simulink model "MultiInverter_StrongGridInstability_Simulation"  (R2020b)
settings: Solver=FixedStepAuto  StartTime=0  StopTime=2  FixedStep=Ts  RelTol=1e-3
undefined symbols (not defined in the file): DeviceDiscreDamping, DevicePara, DeviceType, Fbase, OtherInputs, PowerFlow, Sbase, Ts, Vbase, Wbase, x_e, Ybase, Zbase
libraries: powerlib x61, SimplexPS x21
settings Model: Creator=admin_user  LastModifiedBy=admin_user
settings DataIOCC: ReturnWorkspaceOutputs=off

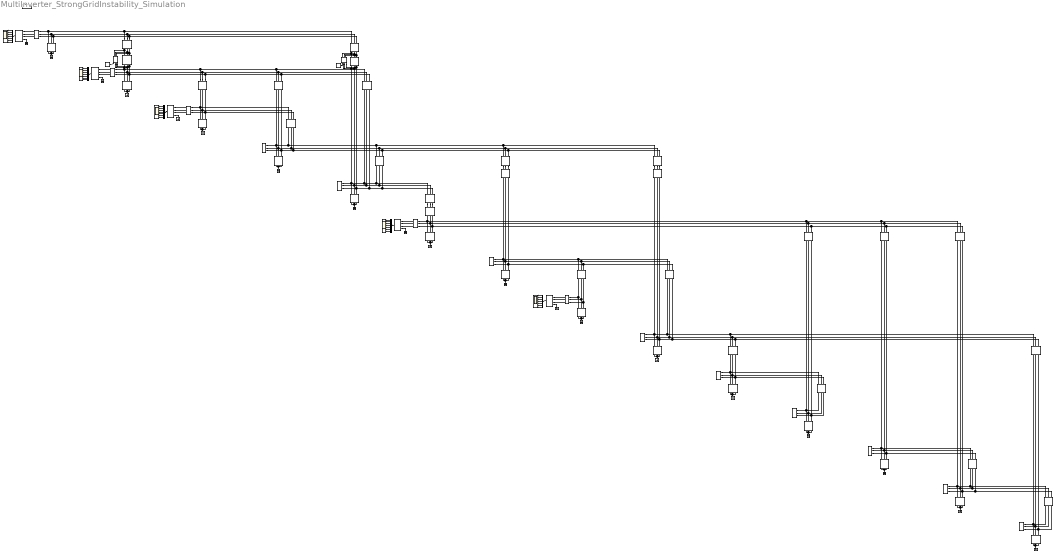
== system MultiInverter_StrongGridInstability_Simulation ==
  B-GND{1,4,8,10,14,16,20,23..24,27,29..30,32,34} (14 alike) : powerlib/Elements/Ground  LConnTagsString=a
  Branch1010 : powerlib/Elements/Three-Phase Parallel RLC Branch  LConnTagsString=A|B|C  RConnTagsString=A|B|C  BranchType=RLC  Resistance=(11.8667)*Zbase  Inductance=(18.4139)*Zbase/Wbase  Capacitance=(1e-05)*Ybase/Wbase  Measurements=None
      settings: SourceProductBaseCode=PS
  Branch1011 : powerlib/Elements/Three-Phase Series RLC Branch  LConnTagsString=A|B|C  RConnTagsString=A|B|C  BranchType=RL  Resistance=(0.08205)*Zbase  Inductance=(0.19207)*Zbase/Wbase  Capacitance=1e-6  Measurements=None
  Branch11 : powerlib/Elements/Three-Phase Parallel RLC Branch  LConnTagsString=A|B|C  RConnTagsString=A|B|C  BranchType=C  Resistance=(Inf)*Zbase  Inductance=1e-3  Capacitance=(0.102)*Ybase/Wbase  Measurements=None
      settings: SourceProductBaseCode=PS
  Branch1111 : powerlib/Elements/Three-Phase Parallel RLC Branch  LConnTagsString=A|B|C  RConnTagsString=A|B|C  BranchType=RLC  Resistance=(31.8511)*Zbase  Inductance=(61.9328)*Zbase/Wbase  Capacitance=(1e-05)*Ybase/Wbase  Measurements=None
      settings: SourceProductBaseCode=PS
  Branch12 : powerlib/Elements/Three-Phase Series RLC Branch  LConnTagsString=A|B|C  RConnTagsString=A|B|C  BranchType=RL  Resistance=(0.01938)*Zbase/5  Inductance=(0.05917)*Zbase/Wbase/5  Capacitance=1e-6  Measurements=None
  Branch1212 : powerlib/Elements/Three-Phase Parallel RLC Branch  LConnTagsString=A|B|C  RConnTagsString=A|B|C  BranchType=RLC  Resistance=(18.8878)*Zbase  Inductance=(72.0098)*Zbase/Wbase  Capacitance=(1e-05)*Ybase/Wbase  Measurements=None
      settings: SourceProductBaseCode=PS
  Branch1213 : powerlib/Elements/Three-Phase Series RLC Branch  LConnTagsString=A|B|C  RConnTagsString=A|B|C  BranchType=RL  Resistance=(0.22092)*Zbase  Inductance=(0.19988)*Zbase/Wbase  Capacitance=1e-6  Measurements=None
  Branch12_v1 : powerlib/Elements/Three-Phase Series RLC Branch  LConnTagsString=A|B|C  RConnTagsString=A|B|C  BranchType=RL  Resistance=(0.01938)*Zbase/5*4  Inductance=(0.05917)*Zbase/Wbase/5*4  Capacitance=1e-6  Measurements=None
  Branch1313 : powerlib/Elements/Three-Phase Parallel RLC Branch  LConnTagsString=A|B|C  RConnTagsString=A|B|C  BranchType=RLC  Resistance=(8.2956)*Zbase  Inductance=(19.3087)*Zbase/Wbase  Capacitance=(1e-05)*Ybase/Wbase  Measurements=None
      settings: SourceProductBaseCode=PS
  Branch1314 : powerlib/Elements/Three-Phase Series RLC Branch  LConnTagsString=A|B|C  RConnTagsString=A|B|C  BranchType=RL  Resistance=(0.17093)*Zbase  Inductance=(0.34802)*Zbase/Wbase  Capacitance=1e-6  Measurements=None
  Branch1414 : powerlib/Elements/Three-Phase Parallel RLC Branch  LConnTagsString=A|B|C  RConnTagsString=A|B|C  BranchType=RLC  Resistance=(7.0495)*Zbase  Inductance=(21.0075)*Zbase/Wbase  Capacitance=(1e-05)*Ybase/Wbase  Measurements=None
      settings: SourceProductBaseCode=PS
  Branch15 : powerlib/Elements/Three-Phase Series RLC Branch  LConnTagsString=A|B|C  RConnTagsString=A|B|C  BranchType=RL  Resistance=(0.05403)*Zbase/5  Inductance=(0.22304)*Zbase/Wbase/5  Capacitance=1e-6  Measurements=None
  Branch15_v1 : powerlib/Elements/Three-Phase Series RLC Branch  LConnTagsString=A|B|C  RConnTagsString=A|B|C  BranchType=RL  Resistance=(0.05403)*Zbase/5*4  Inductance=(0.22304)*Zbase/Wbase/5*4  Capacitance=1e-6  Measurements=None
  Branch22 : powerlib/Elements/Three-Phase Parallel RLC Branch  LConnTagsString=A|B|C  RConnTagsString=A|B|C  BranchType=RLC  Resistance=(5.0324)*Zbase  Inductance=(8.5986)*Zbase/Wbase  Capacitance=(0.1652)*Ybase/Wbase  Measurements=None
      settings: SourceProductBaseCode=PS
  Branch23 : powerlib/Elements/Three-Phase Series RLC Branch  LConnTagsString=A|B|C  RConnTagsString=A|B|C  BranchType=RL  Resistance=(0.04699)*Zbase  Inductance=(0.19797)*Zbase/Wbase  Capacitance=1e-6  Measurements=None
  Branch24 : powerlib/Elements/Three-Phase Series RLC Branch  LConnTagsString=A|B|C  RConnTagsString=A|B|C  BranchType=RL  Resistance=(0.05811)*Zbase  Inductance=(0.17632)*Zbase/Wbase  Capacitance=1e-6  Measurements=None
  Branch25 : powerlib/Elements/Three-Phase Series RLC Branch  LConnTagsString=A|B|C  RConnTagsString=A|B|C  BranchType=RL  Resistance=(0.05695)*Zbase  Inductance=(0.17388)*Zbase/Wbase  Capacitance=1e-6  Measurements=None
  Branch33 : powerlib/Elements/Three-Phase Parallel RLC Branch  LConnTagsString=A|B|C  RConnTagsString=A|B|C  BranchType=RLC  Resistance=(1.0829)*Zbase  Inductance=(5.3689)*Zbase/Wbase  Capacitance=(0.0566)*Ybase/Wbase  Measurements=None
      settings: SourceProductBaseCode=PS
  Branch34 : powerlib/Elements/Three-Phase Series RLC Branch  LConnTagsString=A|B|C  RConnTagsString=A|B|C  BranchType=RL  Resistance=(0.06701)*Zbase  Inductance=(0.17103)*Zbase/Wbase  Capacitance=1e-6  Measurements=None
  Branch44 : powerlib/Elements/Three-Phase Parallel RLC Branch  LConnTagsString=A|B|C  RConnTagsString=A|B|C  BranchType=RC  Resistance=(2.196)*Zbase  Inductance=1e-3  Capacitance=(0.083954)*Ybase/Wbase  Measurements=None
      settings: SourceProductBaseCode=PS
  Branch45 : powerlib/Elements/Three-Phase Series RLC Branch  LConnTagsString=A|B|C  RConnTagsString=A|B|C  BranchType=RL  Resistance=(0.01335)*Zbase  Inductance=(0.04211)*Zbase/Wbase  Capacitance=1e-6  Measurements=None
  Branch47 : powerlib/Elements/Three-Phase Series RLC Branch  LConnTagsString=A|B|C  RConnTagsString=A|B|C  BranchType=RL  Resistance=(0.020912)*Zbase  Inductance=(0.20912)*Zbase/Wbase  Capacitance=1e-6  Measurements=None
  Branch49 : powerlib/Elements/Three-Phase Series RLC Branch  LConnTagsString=A|B|C  RConnTagsString=A|B|C  BranchType=RL  Resistance=(0.055618)*Zbase  Inductance=(0.55618)*Zbase/Wbase  Capacitance=1e-6  Measurements=None
  Branch55 : powerlib/Elements/Three-Phase Parallel RLC Branch  LConnTagsString=A|B|C  RConnTagsString=A|B|C  BranchType=RLC  Resistance=(13.9338)*Zbase  Inductance=(66.1856)*Zbase/Wbase  Capacitance=(0.0838)*Ybase/Wbase  Measurements=None
      settings: SourceProductBaseCode=PS
  Branch56 : powerlib/Elements/Three-Phase Series RLC Branch  LConnTagsString=A|B|C  RConnTagsString=A|B|C  BranchType=RL  Resistance=(0.025202)*Zbase  Inductance=(0.25202)*Zbase/Wbase  Capacitance=1e-6  Measurements=None
  Branch611 : powerlib/Elements/Three-Phase Series RLC Branch  LConnTagsString=A|B|C  RConnTagsString=A|B|C  BranchType=RL  Resistance=(0.09498)*Zbase  Inductance=(0.1989)*Zbase/Wbase  Capacitance=1e-6  Measurements=None
  Branch612 : powerlib/Elements/Three-Phase Series RLC Branch  LConnTagsString=A|B|C  RConnTagsString=A|B|C  BranchType=RL  Resistance=(0.12291)*Zbase  Inductance=(0.25581)*Zbase/Wbase  Capacitance=1e-6  Measurements=None
  Branch613 : powerlib/Elements/Three-Phase Series RLC Branch  LConnTagsString=A|B|C  RConnTagsString=A|B|C  BranchType=RL  Resistance=(0.06615)*Zbase  Inductance=(0.13027)*Zbase/Wbase  Capacitance=1e-6  Measurements=None
  Branch66 : powerlib/Elements/Three-Phase Parallel RLC Branch  LConnTagsString=A|B|C  RConnTagsString=A|B|C  BranchType=RLC  Resistance=(10.2223)*Zbase  Inductance=(15.2653)*Zbase/Wbase  Capacitance=(1e-05)*Ybase/Wbase  Measurements=None
      settings: SourceProductBaseCode=PS
  Branch77 : powerlib/Elements/Three-Phase Parallel RLC Branch  LConnTagsString=A|B|C  RConnTagsString=A|B|C  BranchType=C  Resistance=(Inf)*Zbase  Inductance=1e-3  Capacitance=(1e-05)*Ybase/Wbase  Measurements=None
      settings: SourceProductBaseCode=PS
  Branch78 : powerlib/Elements/Three-Phase Series RLC Branch  LConnTagsString=A|B|C  RConnTagsString=A|B|C  BranchType=RL  Resistance=(0.017615)*Zbase  Inductance=(0.17615)*Zbase/Wbase  Capacitance=1e-6  Measurements=None
  Branch79 : powerlib/Elements/Three-Phase Series RLC Branch  LConnTagsString=A|B|C  RConnTagsString=A|B|C  BranchType=RL  Resistance=(0.011001)*Zbase  Inductance=(0.11001)*Zbase/Wbase  Capacitance=1e-6  Measurements=None
  Branch88 : powerlib/Elements/Three-Phase Parallel RLC Branch  LConnTagsString=A|B|C  RConnTagsString=A|B|C  BranchType=C  Resistance=(Inf)*Zbase  Inductance=1e-3  Capacitance=(1e-05)*Ybase/Wbase  Measurements=None
      settings: SourceProductBaseCode=PS
  Branch910 : powerlib/Elements/Three-Phase Series RLC Branch  LConnTagsString=A|B|C  RConnTagsString=A|B|C  BranchType=RL  Resistance=(0.03181)*Zbase  Inductance=(0.0845)*Zbase/Wbase  Capacitance=1e-6  Measurements=None
  Branch914 : powerlib/Elements/Three-Phase Series RLC Branch  LConnTagsString=A|B|C  RConnTagsString=A|B|C  BranchType=RL  Resistance=(0.12711)*Zbase  Inductance=(0.27038)*Zbase/Wbase  Capacitance=1e-6  Measurements=None
  Branch99 : powerlib/Elements/Three-Phase Parallel RLC Branch  LConnTagsString=A|B|C  RConnTagsString=A|B|C  BranchType=RLC  Resistance=(3.6116)*Zbase  Inductance=(6.4182)*Zbase/Wbase  Capacitance=(1e-05)*Ybase/Wbase  Measurements=None
      settings: SourceProductBaseCode=PS
  Bus{1..14} (14 alike) : SimplexPS/Three-Phase Bus  Vbase=1  Sbase=1
      settings: SourceProductName=Simplex Power Systems
  D-GND{1..3,6,8} (5 alike) : powerlib/Elements/Ground  LConnTagsString=a
  D-Scope{1..3,6,8} (5 alike) : Scope  NumInputPorts=7
  DS-Bus{1..3,6,8} (5 alike) : BusSelector  OutputSignals=v_dq,i_dq,v_abc,i_abc,w,theta,pq
  Single Pulse : SimplexPS/Single Pulse  t0=1  dt=0.4  Am=1
      settings: SourceProductName=Simplex Power Systems
  Single Pulse1 : SimplexPS/Single Pulse  t0=1  dt=0.4  Am=1
      settings: SourceProductName=Simplex Power Systems
  Three-Phase Breaker : powerlib/Elements/Three-Phase Breaker  InitialState=open  SwitchA=on  SwitchB=on  SwitchC=on  SwitchTimes="[1/60  5/60]"  External=on  BreakerResistance=0.01  SnubberResistance=1e6  SnubberCapacitance=inf  Measurements=None
  Three-Phase Breaker1 : powerlib/Elements/Three-Phase Breaker  InitialState=open  SwitchA=on  SwitchB=on  SwitchC=on  SwitchTimes="[1/60  5/60]"  External=on  BreakerResistance=0.01  SnubberResistance=1e6  SnubberCapacitance=inf  Measurements=None
  Transformer47 : powerlib/Elements/Three-Phase Transformer (Two Windings)  Winding1Connection=Yg  Winding2Connection=Yg  CoreType=Three single-phase transformers  SetSaturation=off  Hysteresis=off  DataFile='hysteresis'  SetInitialFlux=off  Measurements=None  UNITS=pu  NominalPower=[Sbase, Fbase]  Winding1=[0.978*Vbase, 0, 0]  Winding2=[Vbase, 0, 0]  Rm=1e4  Lm=1e4  L0=0.5  Saturation=[ 0,0 ; 0.0024,1.2 ; 1.0,1.52 ]  InitialFluxes=[ 0.8 , -0.8 , 0.7 ]  BreakLoop=off  DiscreteSolver=Trapezoidal iterative  DataType=off  TransfoNumber=1
  Transformer49 : powerlib/Elements/Three-Phase Transformer (Two Windings)  Winding1Connection=Yg  Winding2Connection=Yg  CoreType=Three single-phase transformers  SetSaturation=off  Hysteresis=off  DataFile='hysteresis'  SetInitialFlux=off  Measurements=None  UNITS=pu  NominalPower=[Sbase, Fbase]  Winding1=[0.969*Vbase, 0, 0]  Winding2=[Vbase, 0, 0]  Rm=1e4  Lm=1e4  L0=0.5  Saturation=[ 0,0 ; 0.0024,1.2 ; 1.0,1.52 ]  InitialFluxes=[ 0.8 , -0.8 , 0.7 ]  BreakLoop=off  DiscreteSolver=Trapezoidal iterative  DataType=off  TransfoNumber=1
  Transformer56 : powerlib/Elements/Three-Phase Transformer (Two Windings)  Winding1Connection=Yg  Winding2Connection=Yg  CoreType=Three single-phase transformers  SetSaturation=off  Hysteresis=off  DataFile='hysteresis'  SetInitialFlux=off  Measurements=None  UNITS=pu  NominalPower=[Sbase, Fbase]  Winding1=[0.932*Vbase, 0, 0]  Winding2=[Vbase, 0, 0]  Rm=1e4  Lm=1e4  L0=0.5  Saturation=[ 0,0 ; 0.0024,1.2 ; 1.0,1.52 ]  InitialFluxes=[ 0.8 , -0.8 , 0.7 ]  BreakLoop=off  DiscreteSolver=Trapezoidal iterative  DataType=off  TransfoNumber=1
  VSI-Droop1 : SimplexPS/Grid-Forming Voltage-Source Inverter (dq-Frame System Object)  Ts=Ts  Sbase=Sbase  Vbase=Vbase  Wbase=Wbase  DeviceType=DeviceType{1}  DevicePara=DevicePara{1}  PowerFlow=PowerFlow{1}  x0=x_e{1}  OtherInputs=OtherInputs{1}  DiscreMethod=Hybrid Trapezoidal  EnableInsideModification=off  DiscreDampingFlag=on  DiscreDampingValue=DeviceDiscreDamping{1}  LinearizationTimes=1  DirectFeedthrough=off
      settings: SourceProductName=Simplex Power Systems
  VSI-Droop3 : SimplexPS/Grid-Forming Voltage-Source Inverter (dq-Frame System Object)  Ts=Ts  Sbase=Sbase  Vbase=Vbase  Wbase=Wbase  DeviceType=DeviceType{3}  DevicePara=DevicePara{3}  PowerFlow=PowerFlow{3}  x0=x_e{3}  OtherInputs=OtherInputs{3}  DiscreMethod=Hybrid Trapezoidal  EnableInsideModification=off  DiscreDampingFlag=on  DiscreDampingValue=DeviceDiscreDamping{3}  LinearizationTimes=1  DirectFeedthrough=off
      settings: SourceProductName=Simplex Power Systems
  VSI-Droop6 : SimplexPS/Grid-Forming Voltage-Source Inverter (dq-Frame System Object)  Ts=Ts  Sbase=Sbase  Vbase=Vbase  Wbase=Wbase  DeviceType=DeviceType{6}  DevicePara=DevicePara{6}  PowerFlow=PowerFlow{6}  x0=x_e{6}  OtherInputs=OtherInputs{6}  DiscreMethod=Hybrid Trapezoidal  EnableInsideModification=off  DiscreDampingFlag=on  DiscreDampingValue=DeviceDiscreDamping{6}  LinearizationTimes=1  DirectFeedthrough=off
      settings: SourceProductName=Simplex Power Systems
  VSI-PLL2 : SimplexPS/Grid-Following Voltage-Source Inverter (dq-Frame System Object)  Ts=Ts  Sbase=Sbase  Vbase=Vbase  Wbase=Wbase  DeviceType=DeviceType{2}  DevicePara=DevicePara{2}  PowerFlow=PowerFlow{2}  x0=x_e{2}  OtherInputs=OtherInputs{2}  DiscreMethod=Hybrid Trapezoidal  EnableInsideModification=off  DiscreDampingFlag=on  DiscreDampingValue=DeviceDiscreDamping{2}  LinearizationTimes=1  DirectFeedthrough=off
      settings: SourceProductName=Simplex Power Systems
  VSI-PLL8 : SimplexPS/Grid-Following Voltage-Source Inverter (dq-Frame System Object)  Ts=Ts  Sbase=Sbase  Vbase=Vbase  Wbase=Wbase  DeviceType=DeviceType{8}  DevicePara=DevicePara{8}  PowerFlow=PowerFlow{8}  x0=x_e{8}  OtherInputs=OtherInputs{8}  DiscreMethod=Hybrid Trapezoidal  EnableInsideModification=off  DiscreDampingFlag=on  DiscreDampingValue=DeviceDiscreDamping{8}  LinearizationTimes=1  DirectFeedthrough=off
      settings: SourceProductName=Simplex Power Systems
  powergui : powerlib/powergui  Priority=1  SimulationMode=Discrete  SampleTime=Ts  frequency=60  Iterations=50  frequencyindice=0  Pbase=100e6  ErrMax=1e-4  UnitsV=kV  UnitsW=MW  buscounter=0  FunctionMessages=off  echomessages=off  EnableUseOfTLC=off  CurrentSourceSwitches=off  DisableSnubberDevices=off  DisableRonSwitches=off  DisableVfSwitches=off  DisplayEquations=off  AutomaticDiscreteSolvers=off  SolverType=Tustin/Backward Euler (TBE)  Interpol=off  ExternalGateDelay=off  methode=off  Ts=100  x0status=blocks  SPID=on  SwTol=0  HookPort=off  NonlinearTolerance=1e-4  nMaxIteration=100  ContinueOnMaxIteration=off  RestoreLinks=warning  ResistiveCurrentMeasurement=off  Frange=[0:2:500]  Ylog=off  Xlog=on  ShowGrid=off  save=off  variable=ZData  structure=0  ZoomFFT=off  StartTime=0.0  cycles=1  DisplayStyle=1  fundamental=60  FreqAxis=off  MaxFrequency=1000  frequencyindicesteady=1  RmsSteady=1  display=off
  wires:
  VSI-Droop1/1 -> DS-Bus1/1
  DS-Bus1/1 -> D-Scope1/1  "<v_dq>"
  DS-Bus1/2 -> D-Scope1/2  "<i_dq>"
  DS-Bus1/3 -> D-Scope1/3  "<v_abc>"
  DS-Bus1/4 -> D-Scope1/4  "<i_abc>"
  DS-Bus1/5 -> D-Scope1/5  "<w>"
  DS-Bus1/6 -> D-Scope1/6  "<theta>"
  DS-Bus1/7 -> D-Scope1/7  "<pq>"
  VSI-PLL2/1 -> DS-Bus2/1
  DS-Bus2/1 -> D-Scope2/1  "<v_dq>"
  DS-Bus2/2 -> D-Scope2/2  "<i_dq>"
  DS-Bus2/3 -> D-Scope2/3  "<v_abc>"
  DS-Bus2/4 -> D-Scope2/4  "<i_abc>"
  DS-Bus2/5 -> D-Scope2/5  "<w>"
  DS-Bus2/6 -> D-Scope2/6  "<theta>"
  DS-Bus2/7 -> D-Scope2/7  "<pq>"
  VSI-Droop3/1 -> DS-Bus3/1
  DS-Bus3/1 -> D-Scope3/1  "<v_dq>"
  DS-Bus3/2 -> D-Scope3/2  "<i_dq>"
  DS-Bus3/3 -> D-Scope3/3  "<v_abc>"
  DS-Bus3/4 -> D-Scope3/4  "<i_abc>"
  DS-Bus3/5 -> D-Scope3/5  "<w>"
  DS-Bus3/6 -> D-Scope3/6  "<theta>"
  DS-Bus3/7 -> D-Scope3/7  "<pq>"
  VSI-Droop6/1 -> DS-Bus6/1
  DS-Bus6/1 -> D-Scope6/1  "<v_dq>"
  DS-Bus6/2 -> D-Scope6/2  "<i_dq>"
  DS-Bus6/3 -> D-Scope6/3  "<v_abc>"
  DS-Bus6/4 -> D-Scope6/4  "<i_abc>"
  DS-Bus6/5 -> D-Scope6/5  "<w>"
  DS-Bus6/6 -> D-Scope6/6  "<theta>"
  DS-Bus6/7 -> D-Scope6/7  "<pq>"
  VSI-PLL8/1 -> DS-Bus8/1
  DS-Bus8/1 -> D-Scope8/1  "<v_dq>"
  DS-Bus8/2 -> D-Scope8/2  "<i_dq>"
  DS-Bus8/3 -> D-Scope8/3  "<v_abc>"
  DS-Bus8/4 -> D-Scope8/4  "<i_abc>"
  DS-Bus8/5 -> D-Scope8/5  "<w>"
  DS-Bus8/6 -> D-Scope8/6  "<theta>"
  DS-Bus8/7 -> D-Scope8/7  "<pq>"
  Single Pulse/1 -> Three-Phase Breaker/1
  Single Pulse1/1 -> Three-Phase Breaker1/1
  connections:
  VSI-Droop1/LConn1 -- Bus1/LConn1
  VSI-Droop1/LConn2 -- Bus1/LConn2
  VSI-Droop1/LConn3 -- Bus1/LConn3
  VSI-PLL2/LConn1 -- Bus2/LConn1
  VSI-PLL2/LConn2 -- Bus2/LConn2
  VSI-PLL2/LConn3 -- Bus2/LConn3
  VSI-Droop3/LConn1 -- Bus3/LConn1
  VSI-Droop3/LConn2 -- Bus3/LConn2
  VSI-Droop3/LConn3 -- Bus3/LConn3
  VSI-Droop6/LConn1 -- Bus6/LConn1
  VSI-Droop6/LConn2 -- Bus6/LConn2
  VSI-Droop6/LConn3 -- Bus6/LConn3
  VSI-PLL8/LConn1 -- Bus8/LConn1
  VSI-PLL8/LConn2 -- Bus8/LConn2
  VSI-PLL8/LConn3 -- Bus8/LConn3
  VSI-Droop1/LConn4 -- D-GND1/LConn1
  VSI-PLL2/LConn4 -- D-GND2/LConn1
  VSI-Droop3/LConn4 -- D-GND3/LConn1
  VSI-Droop6/LConn4 -- D-GND6/LConn1
  VSI-PLL8/LConn4 -- D-GND8/LConn1
  Branch11/RConn1 -- Branch11/RConn2 -- Branch11/RConn3 -- B-GND1/LConn1
  Branch22/RConn1 -- Branch22/RConn2 -- Branch22/RConn3 -- B-GND4/LConn1
  Branch33/RConn1 -- Branch33/RConn2 -- Branch33/RConn3 -- B-GND8/LConn1
  Branch44/RConn1 -- Branch44/RConn2 -- Branch44/RConn3 -- B-GND10/LConn1
  Branch55/RConn1 -- Branch55/RConn2 -- Branch55/RConn3 -- B-GND14/LConn1
  Branch66/RConn1 -- Branch66/RConn2 -- Branch66/RConn3 -- B-GND16/LConn1
  Branch77/RConn1 -- Branch77/RConn2 -- Branch77/RConn3 -- B-GND20/LConn1
  Branch88/RConn1 -- Branch88/RConn2 -- Branch88/RConn3 -- B-GND23/LConn1
  Branch99/RConn1 -- Branch99/RConn2 -- Branch99/RConn3 -- B-GND24/LConn1
  Branch1010/RConn1 -- Branch1010/RConn2 -- Branch1010/RConn3 -- B-GND27/LConn1
  Branch1111/RConn1 -- Branch1111/RConn2 -- Branch1111/RConn3 -- B-GND29/LConn1
  Branch1212/RConn1 -- Branch1212/RConn2 -- Branch1212/RConn3 -- B-GND30/LConn1
  Branch1313/RConn1 -- Branch1313/RConn2 -- Branch1313/RConn3 -- B-GND32/LConn1
  Branch1414/RConn1 -- Branch1414/RConn2 -- Branch1414/RConn3 -- B-GND34/LConn1
  Branch23/LConn1 -- Branch25/LConn1 -- Branch24/LConn1 -- Three-Phase Breaker/LConn1 -- Branch12_v1/RConn1 -- Branch22/LConn1 -- Bus2/RConn1
  Branch23/LConn2 -- Branch25/LConn2 -- Branch24/LConn2 -- Branch12_v1/RConn2 -- Three-Phase Breaker/LConn2 -- Branch22/LConn2 -- Bus2/RConn2
  Branch23/LConn3 -- Branch25/LConn3 -- Branch24/LConn3 -- Three-Phase Breaker/LConn3 -- Branch12_v1/RConn3 -- Bus2/RConn3 -- Branch22/LConn3
  Branch12/LConn1 -- Bus1/RConn1 -- Branch11/LConn1 -- Branch15/LConn1
  Branch12/LConn2 -- Bus1/RConn2 -- Branch11/LConn2 -- Branch15/LConn2
  Branch12/LConn3 -- Bus1/RConn3 -- Branch11/LConn3 -- Branch15/LConn3
  Branch25/RConn1 -- Three-Phase Breaker1/LConn1 -- Branch15_v1/RConn1 -- Bus5/RConn1 -- Branch55/LConn1 -- Transformer56/LConn1 -- Branch45/RConn1
  Branch25/RConn2 -- Transformer56/LConn2 -- Branch45/RConn2 -- Three-Phase Breaker1/LConn2 -- Branch15_v1/RConn2 -- Bus5/RConn2 -- Branch55/LConn2
  Branch25/RConn3 -- Transformer56/LConn3 -- Branch45/RConn3 -- Three-Phase Breaker1/LConn3 -- Branch15_v1/RConn3 -- Bus5/RConn3 -- Branch55/LConn3
  Branch23/RConn1 -- Bus3/RConn1 -- Branch33/LConn1 -- Branch34/LConn1
  Branch23/RConn2 -- Bus3/RConn2 -- Branch33/LConn2 -- Branch34/LConn2
  Branch23/RConn3 -- Bus3/RConn3 -- Branch33/LConn3 -- Branch34/LConn3
  Branch24/RConn1 -- Bus4/RConn1 -- Branch44/LConn1 -- Transformer49/LConn1 -- Transformer47/LConn1 -- Branch45/LConn1 -- Branch34/RConn1
  Branch24/RConn2 -- Bus4/RConn2 -- Branch44/LConn2 -- Transformer49/LConn2 -- Transformer47/LConn2 -- Branch45/LConn2 -- Branch34/RConn2
  Branch24/RConn3 -- Bus4/RConn3 -- Branch44/LConn3 -- Transformer49/LConn3 -- Transformer47/LConn3 -- Branch45/LConn3 -- Branch34/RConn3
  Branch47/RConn1 -- Bus7/RConn1 -- Branch77/LConn1 -- Branch79/LConn1 -- Branch78/LConn1
  Branch47/RConn2 -- Bus7/RConn2 -- Branch77/LConn2 -- Branch79/LConn2 -- Branch78/LConn2
  Branch47/RConn3 -- Bus7/RConn3 -- Branch77/LConn3 -- Branch79/LConn3 -- Branch78/LConn3
  Transformer47/RConn1 -- Branch47/LConn1
  Transformer47/RConn2 -- Branch47/LConn2
  Transformer47/RConn3 -- Branch47/LConn3
  Branch49/RConn1 -- Bus9/RConn1 -- Branch99/LConn1 -- Branch914/LConn1 -- Branch910/LConn1 -- Branch79/RConn1
  Branch49/RConn2 -- Bus9/RConn2 -- Branch99/LConn2 -- Branch914/LConn2 -- Branch910/LConn2 -- Branch79/RConn2
  Branch49/RConn3 -- Bus9/RConn3 -- Branch99/LConn3 -- Branch914/LConn3 -- Branch910/LConn3 -- Branch79/RConn3
  Transformer49/RConn1 -- Branch49/LConn1
  Transformer49/RConn2 -- Branch49/LConn2
  Transformer49/RConn3 -- Branch49/LConn3
  Branch56/RConn1 -- Bus6/RConn1 -- Branch66/LConn1 -- Branch613/LConn1 -- Branch612/LConn1 -- Branch611/LConn1
  Branch56/RConn2 -- Bus6/RConn2 -- Branch66/LConn2 -- Branch613/LConn2 -- Branch612/LConn2 -- Branch611/LConn2
  Branch56/RConn3 -- Bus6/RConn3 -- Branch66/LConn3 -- Branch613/LConn3 -- Branch612/LConn3 -- Branch611/LConn3
  Transformer56/RConn1 -- Branch56/LConn1
  Transformer56/RConn2 -- Branch56/LConn2
  Transformer56/RConn3 -- Branch56/LConn3
  Branch611/RConn1 -- Bus11/RConn1 -- Branch1111/LConn1 -- Branch1011/RConn1
  Branch611/RConn2 -- Bus11/RConn2 -- Branch1111/LConn2 -- Branch1011/RConn2
  Branch611/RConn3 -- Bus11/RConn3 -- Branch1111/LConn3 -- Branch1011/RConn3
  Branch612/RConn1 -- Bus12/RConn1 -- Branch1212/LConn1 -- Branch1213/LConn1
  Branch612/RConn2 -- Bus12/RConn2 -- Branch1212/LConn2 -- Branch1213/LConn2
  Branch612/RConn3 -- Bus12/RConn3 -- Branch1212/LConn3 -- Branch1213/LConn3
  Branch613/RConn1 -- Bus13/RConn1 -- Branch1313/LConn1 -- Branch1314/LConn1 -- Branch1213/RConn1
  Branch613/RConn2 -- Bus13/RConn2 -- Branch1313/LConn2 -- Branch1314/LConn2 -- Branch1213/RConn2
  Branch613/RConn3 -- Bus13/RConn3 -- Branch1313/LConn3 -- Branch1314/LConn3 -- Branch1213/RConn3
  Branch78/RConn1 -- Bus8/RConn1 -- Branch88/LConn1
  Branch78/RConn2 -- Bus8/RConn2 -- Branch88/LConn2
  Branch78/RConn3 -- Bus8/RConn3 -- Branch88/LConn3
  Branch910/RConn1 -- Bus10/RConn1 -- Branch1010/LConn1 -- Branch1011/LConn1
  Branch910/RConn2 -- Bus10/RConn2 -- Branch1010/LConn2 -- Branch1011/LConn2
  Branch910/RConn3 -- Bus10/RConn3 -- Branch1010/LConn3 -- Branch1011/LConn3
  Branch914/RConn1 -- Bus14/RConn1 -- Branch1414/LConn1 -- Branch1314/RConn1
  Branch914/RConn2 -- Bus14/RConn2 -- Branch1414/LConn2 -- Branch1314/RConn2
  Branch914/RConn3 -- Bus14/RConn3 -- Branch1414/LConn3 -- Branch1314/RConn3
  Branch12_v1/LConn1 -- Three-Phase Breaker/RConn1 -- Branch12/RConn1
  Branch12_v1/LConn3 -- Three-Phase Breaker/RConn3 -- Branch12/RConn3
  Branch12_v1/LConn2 -- Three-Phase Breaker/RConn2 -- Branch12/RConn2
  Branch15_v1/LConn1 -- Three-Phase Breaker1/RConn1 -- Branch15/RConn1
  Branch15_v1/LConn2 -- Three-Phase Breaker1/RConn2 -- Branch15/RConn2
  Branch15_v1/LConn3 -- Branch15/RConn3 -- Three-Phase Breaker1/RConn3
